simulink model "PI_Controller"  (R2023a)
settings: Solver=VariableStepAuto  StartTime=0.0  StopTime=10.0  RelTol=1e-3
undefined symbols (not defined in the file or in its folder): a, b, K, r, z_PI
settings Model: Creator=m260477  LastModifiedBy=m260477

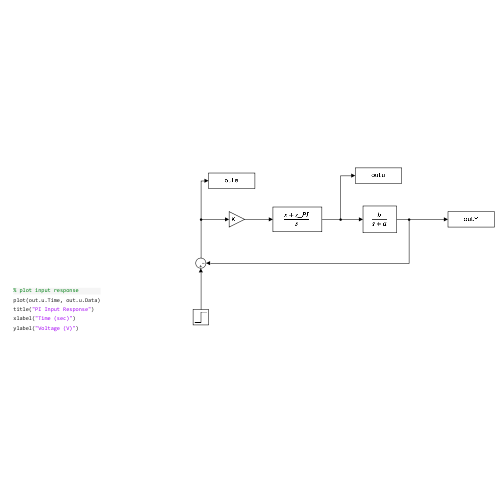
[thumbnail: Simulink's stored preview of the top-level diagram]
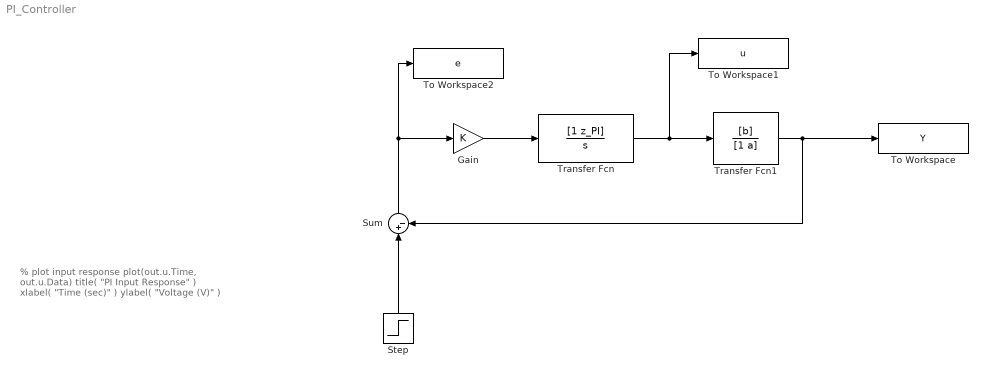
== system PI_Controller ==
  note: % plot input response
      | plot(out.u.Time, out.u.Data)
      | title( "PI Input Response" )
      | xlabel( "Time (sec)" )
      | ylabel( "Voltage (V)" )
  Gain : Gain  Gain=K
  Step : Step  Time=0  After=r  SampleTime=0
  Sum : Sum  Inputs=|+-
  To Workspace : ToWorkspace  VariableName=Y  SaveFormat=Timeseries  SampleTime=-1
  To Workspace1 : ToWorkspace  VariableName=u  SaveFormat=Timeseries  SampleTime=-1
  To Workspace2 : ToWorkspace  VariableName=e  SaveFormat=Timeseries  SampleTime=-1
  Transfer Fcn : TransferFcn  Numerator=[1 z_PI]  Denominator=[1 0]
  Transfer Fcn1 : TransferFcn  Numerator=[b]  Denominator=[1 a]
  wires:
  Gain/1 -> Transfer Fcn/1
  Sum/1 -> To Workspace2/1, Gain/1
  Transfer Fcn/1 -> To Workspace1/1, Transfer Fcn1/1
  Transfer Fcn1/1 -> To Workspace/1, Sum/2
  Step/1 -> Sum/1
